simulink model "simulation"  (R2025b)
settings: Solver=VariableStepAuto  StartTime=0.0  StopTime=10.0  RelTol=1e-3
settings Model: Creator=dhruva  LastModifiedBy=dhruv
settings RTWCC: GPUComputeCapability=3.5

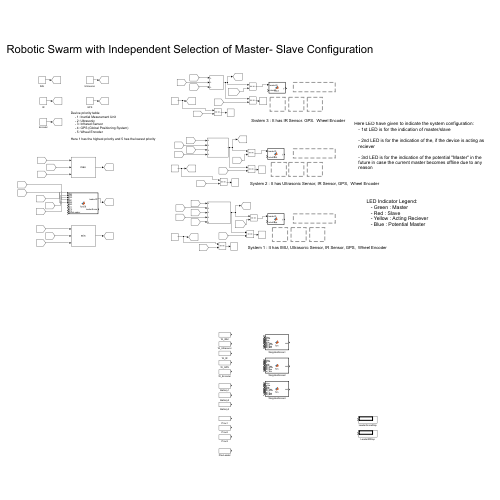
[thumbnail: Simulink's stored preview of the top-level diagram]
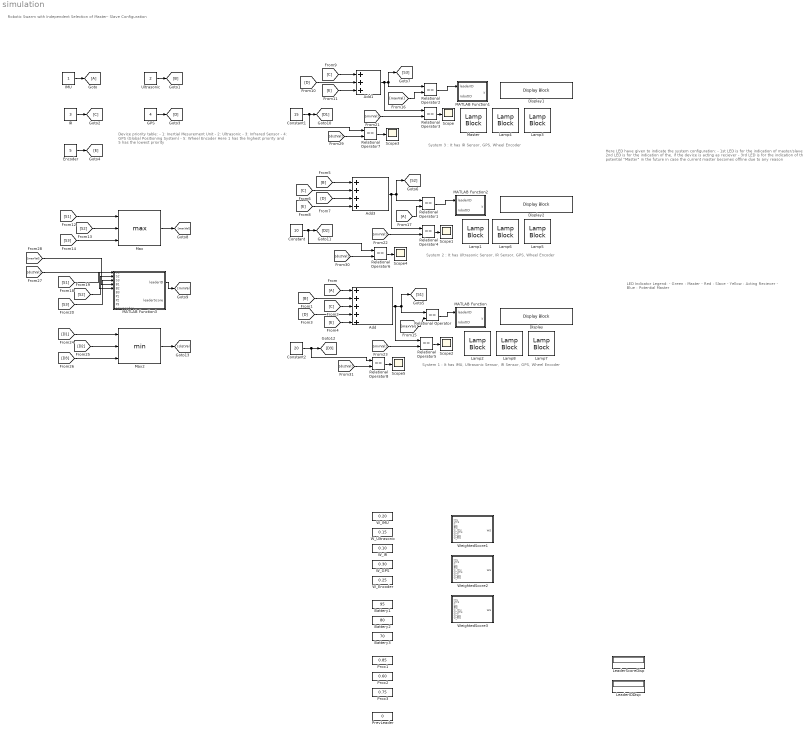
== system simulation ==
  note: LED Indicator Legend:
      | - Green : Master
      | - Red : Slave
      | - Yellow : Acting Reciever
      | - Blue : Potential Master
  note: Here LED have given to indicate the system configuration:
      | - 1st LED is for the indication of master/slave
      |
      | - 2nd LED is for the indication of the, if the device is acting as reciever
      |
      | - 3rd LED is for the indication of the potential "Master" in the future in case the current master becomes offline due to any reason
  note: System 1 : It has IMU, Ultrasonic Sensor, IR Sensor, GPS, Wheel Encoder
  note: Device priority table:
      | - 1: Inertial Mesurement Unit
      | - 2: Ultrasonic
      | - 3: Infrared Sensor
      | - 4: GPS (Global Positioning System)
      | - 5: Wheel Encoder
      |
      | Here 1 has the highest priority and 5 has the lowest priority
  note: Robotic Swarm with Independent Selection of Master- Slave Configuration
  note: System 2 : It has Ultrasonic Sensor, IR Sensor, GPS, Wheel Encoder
  note: System 3 : It has IR Sensor, GPS, Wheel Encoder
  Add : Sum  Inputs=+++++
  Add1 : Sum  Inputs=+++
  Add3 : Sum  Inputs=++++
  Battery1 : Constant  Value=95
  Battery2 : Constant  Value=80
  Battery3 : Constant  Value=70
  Constant : Constant  Value=10
  Constant1 : Constant  Value=15
  Constant2 : Constant  Value=20
  Display : DisplayBlock  LabelPosition=Hide  Transparency=1  GridColor=[0.502, 0.502, 0.502]
  Display1 : DisplayBlock  LabelPosition=Hide  Transparency=1  GridColor=[0.502, 0.502, 0.502]
  Display2 : DisplayBlock  LabelPosition=Hide  Transparency=1  GridColor=[0.502, 0.502, 0.502]
  Encoder : Constant  Value=5
  From : From
  From17 : From
  GPS : Constant  Value=4
  Goto : Goto
  IMU : Constant
  IR : Constant  Value=3
  Lamp{1..8} (8 alike) : LampBlock  LabelPosition=Hide  DefaultColor=[192.0, 192.0, 192.0]
  LeaderIDDisp : Display
  LeaderScoreDisp : Display
  MATLAB Function : MATLAB Function  TreatAsAtomicUnit=on
  MATLAB Function1 : MATLAB Function  TreatAsAtomicUnit=on
  MATLAB Function2 : MATLAB Function  TreatAsAtomicUnit=on
  MATLAB Function3 : MATLAB Function  TreatAsAtomicUnit=on
  Master : LampBlock  LabelPosition=Hide  DefaultColor=[192.0, 192.0, 192.0]
  Max : MinMax  Function=max  Inputs=3
  Max2 : MinMax  Inputs=3
  PrevLeader : Constant  Value=0
  Prox1 : Constant  Value=0.85
  Prox2 : Constant  Value=0.60
  Prox3 : Constant  Value=0.75
  Relational Operator{,1..8} (9 alike) : RelationalOperator  Operator===  OutDataTypeStr=boolean  RndMeth=Simplest  InputSameDT=off
  Scope{,1..5} (6 alike) : Scope
      Scope2 settings: DataLoggingVariableName=ScopeData2
      Scope3 settings: ActiveDisplayYMinimum=-1  ActiveDisplayYMaximum=1  DataLoggingVariableName=ScopeData3
      Scope4 settings: ActiveDisplayYMinimum=0.9  ActiveDisplayYMaximum=1.1  DataLoggingVariableName=ScopeData4
      Scope5 settings: ActiveDisplayYMinimum=-1  ActiveDisplayYMaximum=1  DataLoggingVariableName=ScopeData5
  Ultrasonic : Constant  Value=2
  W_Encoder : Constant  Value=0.25
  W_GPS : Constant  Value=0.30
  W_IMU : Constant  Value=0.20
  W_IR : Constant  Value=0.10
  W_Ultrasonic : Constant  Value=0.15
  WeightedScore1 : MATLAB Function  TreatAsAtomicUnit=on
  WeightedScore2 : MATLAB Function  TreatAsAtomicUnit=on
  WeightedScore3 : MATLAB Function  TreatAsAtomicUnit=on
  wires:
  IMU/1 -> Goto/1
  Ultrasonic/1 -> [B]
  IR/1 -> [C]
  GPS/1 -> [D]
  Encoder/1 -> [E]
  From/1 -> Add/1
  [B] -> Add/2
  [C] -> Add/3
  [D] -> Add/4
  [E] -> Add/5
  [B] -> Add3/1
  [C] -> Add3/2
  [D] -> Add3/3
  [E] -> Add3/4
  [C] -> Add1/1
  [D] -> Add1/2
  [E] -> Add1/3
  Add/1 -> Relational Operator5/1, Relational Operator/1, [S1]
  Add3/1 -> Relational Operator4/1, Relational Operator1/1, [S2]
  Add1/1 -> Relational Operator3/1, Relational Operator2/1, [S3]
  [S1] -> Max/1
  [S2] -> Max/2
  [S3] -> Max/3
  [maxVal] -> Relational Operator/2
  Max/1 -> [maxVal]
  Relational Operator/1 -> MATLAB Function/1(leaderID)
  [maxVal] -> Relational Operator2/2
  Relational Operator2/1 -> MATLAB Function1/1(leaderID)
  From17/1 -> Relational Operator1/2
  Relational Operator1/1 -> MATLAB Function2/1(leaderID)
  Relational Operator4/1 -> Scope1/1
  [minVal] -> Relational Operator3/2
  [minVal] -> Relational Operator4/2
  Relational Operator3/1 -> Scope/1
  [minVal] -> Relational Operator5/2
  Relational Operator5/1 -> Scope2/1
  Constant1/1 -> Relational Operator7/1, [D1]
  Constant/1 -> Relational Operator6/1, [D2]
  Constant2/1 -> Relational Operator8/1, [D3]
  Max2/1 -> [distVal]
  [D3] -> Max2/3
  [D2] -> Max2/2
  [D1] -> Max2/1
  [S3] -> MATLAB Function3/3(S3)
  [S2] -> MATLAB Function3/2(S2)
  [S1] -> MATLAB Function3/1(S1)
  [maxVal] -> MATLAB Function3/4(B1)
  [distVal] -> MATLAB Function3/5(B2)
  MATLAB Function3/1(leaderID) -> [minVal]
  [distVal] -> Relational Operator7/2
  [distVal] -> Relational Operator6/2
  [distVal] -> Relational Operator8/2
  Relational Operator7/1 -> Scope3/1
  Relational Operator6/1 -> Scope4/1
  Relational Operator8/1 -> Scope5/1

== matlab function simulation/MATLAB Function1 ==
  data: leaderID input; y output; robotID input
function y = fcn1(leaderID, robotID)
% Display Master/Slave based on leader election result
if leaderID == robotID
    y = "Master";
else
    y = "Slave";
end

== matlab function simulation/MATLAB Function ==
  data: leaderID input; y output; robotID input
function y = fcn(leaderID, robotID)
% Display Master/Slave based on leader election result
if leaderID == robotID
    y = "Master";
else
    y = "Slave";
end

== matlab function simulation/MATLAB Function2 ==
  data: leaderID input; y output; robotID input
function y = fcn(leaderID, robotID)
% Display Master/Slave based on leader election result
if leaderID == robotID
    y = "Master";
else
    y = "Slave";
end

== matlab function simulation/MATLAB Function3 ==
  data: S1 input; S2 input; S3 input; B1 input; leaderID output; B2 input; B3 input; P1 input; P2 input; P3 input; prevLeader input; leaderScore output
function [leaderID, leaderScore] = fcn56(S1, S2, S3, B1, B2, B3, P1, P2, P3, prevLeader)
% IMPROVED Dynamic Leader Selection Algorithm
% Inputs:
%   S1,S2,S3    - Weighted sensor scores for robots 1,2,3
%   B1,B2,B3    - Battery levels (0-100)
%   P1,P2,P3    - Proximity to centroid (0-1)
%   prevLeader  - Previous leader ID (1,2, or 3)
% Outputs:
%   leaderID    - Selected leader (1,2, or 3)
%   leaderScore - The winning score

% --- Tunable weights ---
alpha = 0.55;  % sensor health weight
beta  = 0.25;  % proximity weight
gamma = 0.20;  % battery weight
tau   = 0.08;  % hysteresis threshold

% --- Composite scores ---
L1 = alpha*S1 + beta*P1 + gamma*(B1/100);
L2 = alpha*S2 + beta*P2 + gamma*(B2/100);
L3 = alpha*S3 + beta*P3 + gamma*(B3/100);

scores = [L1, L2, L3];
[maxScore, candidateID] = max(scores);

% --- Hysteresis: only switch if margin > tau ---
if prevLeader >= 1 && prevLeader <= 3
    currentScore = scores(prevLeader);
    margin = maxScore - currentScore;
    if margin <= tau
        leaderID = prevLeader;
        leaderScore = currentScore;
    else
        leaderID = candidateID;
        leaderScore = maxScore;
    end
else
    leaderID = candidateID;
    leaderScore = maxScore;
end

== matlab function simulation/WeightedScore1 ==
  data: imu input; ws output; ultra input; ir input; gps input; enc input; w_imu input; w_ultra input; w_ir input; w_gps input; w_enc input
function ws = fcn(imu, ultra, ir, gps, enc, w_imu, w_ultra, w_ir, w_gps, w_enc)
% Compute weighted sensor health score
% Each sensor value represents health (0-5 scale), weights sum to 1
total_w = w_imu + w_ultra + w_ir + w_gps + w_enc;
ws = (w_imu*imu + w_ultra*ultra + w_ir*ir + w_gps*gps + w_enc*enc) / total_w;

== matlab function simulation/WeightedScore2 ==
  data: imu input; ws output; ultra input; ir input; gps input; enc input; w_imu input; w_ultra input; w_ir input; w_gps input; w_enc input
function ws = fcn(imu, ultra, ir, gps, enc, w_imu, w_ultra, w_ir, w_gps, w_enc)
% Compute weighted sensor health score
% Each sensor value represents health (0-5 scale), weights sum to 1
total_w = w_imu + w_ultra + w_ir + w_gps + w_enc;
ws = (w_imu*imu + w_ultra*ultra + w_ir*ir + w_gps*gps + w_enc*enc) / total_w;

== matlab function simulation/WeightedScore3 ==
  data: imu input; ws output; ultra input; ir input; gps input; enc input; w_imu input; w_ultra input; w_ir input; w_gps input; w_enc input
function ws = fcn(imu, ultra, ir, gps, enc, w_imu, w_ultra, w_ir, w_gps, w_enc)
% Compute weighted sensor health score
% Each sensor value represents health (0-5 scale), weights sum to 1
total_w = w_imu + w_ultra + w_ir + w_gps + w_enc;
ws = (w_imu*imu + w_ultra*ultra + w_ir*ir + w_gps*gps + w_enc*enc) / total_w;
